simulink model "test3"  (R2024b)
settings: Solver=VariableStepAuto  StartTime=0.0  StopTime=20  RelTol=1e-3
settings Model: Creator=Hosein  LastModifiedBy=Hosein

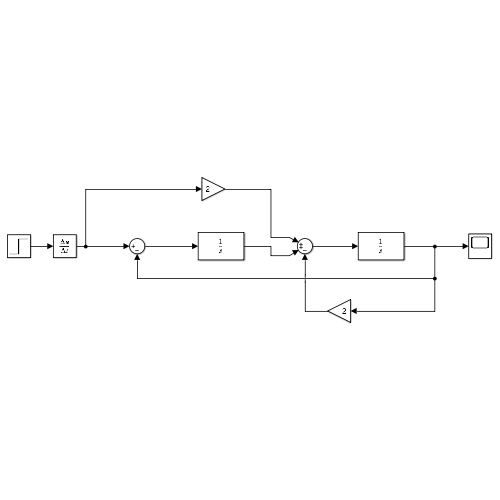
[thumbnail: Simulink's stored preview of the top-level diagram]
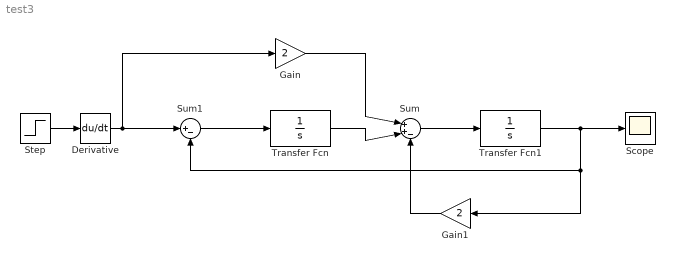
== system test3 ==
  Derivative : Derivative
  Gain : Gain  Gain=2
  Gain1 : Gain  Gain=2
  Scope : Scope
  Step : Step  SampleTime=0
  Sum : Sum  Inputs=|++-
  Sum1 : Sum  Inputs=|+-
  Transfer Fcn : TransferFcn  Denominator=[1 0]
  Transfer Fcn1 : TransferFcn  Denominator=[1 0]
  wires:
  Step/1 -> Derivative/1
  Sum1/1 -> Transfer Fcn/1
  Transfer Fcn1/1 -> Gain1/1, Sum1/2, Scope/1
  Gain1/1 -> Sum/3
  Transfer Fcn/1 -> Sum/2
  Gain/1 -> Sum/1
  Sum/1 -> Transfer Fcn1/1
  Derivative/1 -> Gain/1, Sum1/1
